simulink model "escooter_sequence_diagram_recuperation"  (R2025b)
settings: Solver=VariableStepAuto  StartTime=0.0  StopTime=10.0  RelTol=1e-3
settings Model: Creator=320236370  LastModifiedBy=320236370

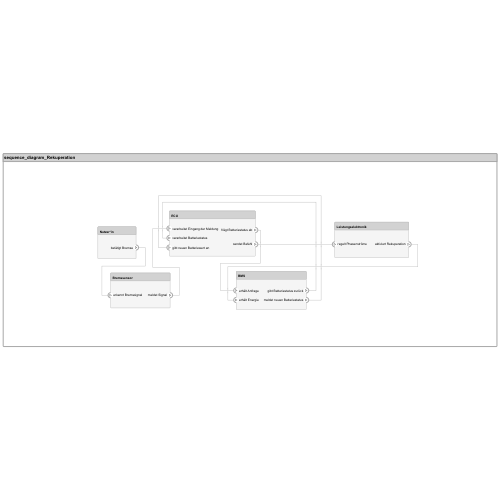
[thumbnail: Simulink's stored preview of the top-level diagram]
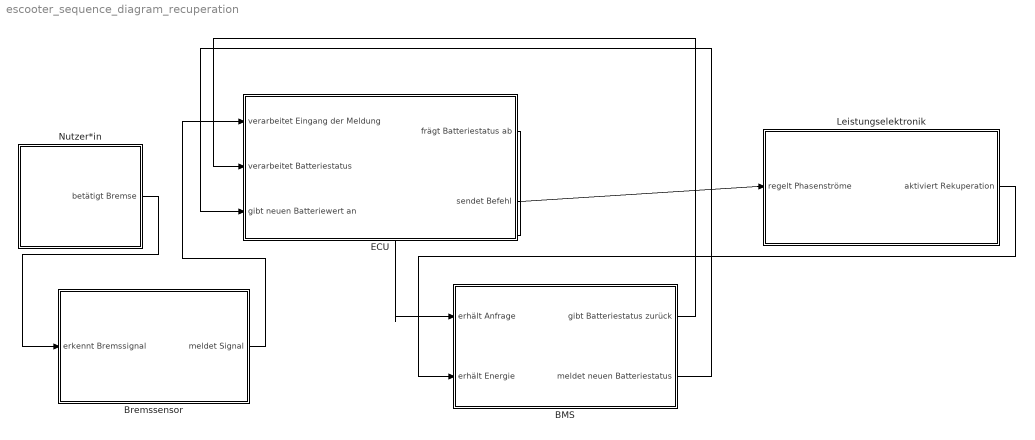
== system escooter_sequence_diagram_recuperation ==
  BMS : Subsystem
      settings: PortSchema="{\"entries\":[{\"content\":{\"headerSize\":26,\"margin\":15,\"minimumSpacing\":25,\"sides\":[{\"content\":{\"connectorIds\":[\"In1\",\"In2\"]},\"type\":\"ConnectorPlacement.EquallySpacedRectSide\",\"uuid\":\"3d49029f-ff69-43f0-9083-eb7baed04898\"},{\"content\":{\"connectorIds\":[\"Out1\",\"Out2\"],\"side\":\"RIGHT\"},\"type\":\"ConnectorPlacement.EquallySpacedRectSide\",\"uuid\":\"1597d90c-c332-40d9-8a70-68f04d256300\"},{\"content\":{\"side\":\"TOP\"},\"type\":\"ConnectorPlacement.EquallySpacedRectSide\",\"uuid\":\"ad895052-9fa6-4dfa-a28f-1843b80a8a3f\"}]},\"type\":\"ConnectorPlacement.EquallySpacedConnector\",\"uuid\":\"8d35fef0-5689-4d8b-850c-97501fa910c2\"}],\"packageUris\":[\"http://schema.mathworks.com/mf0/Connector/R2020b\"],\"version\":\"1.0\"}"
  Bremssensor : Subsystem
      settings: PortSchema="{\"entries\":[{\"content\":{\"headerSize\":26,\"margin\":15,\"minimumSpacing\":25,\"sides\":[{\"content\":{\"connectorIds\":[\"In1\"]},\"type\":\"ConnectorPlacement.EquallySpacedRectSide\",\"uuid\":\"3d49029f-ff69-43f0-9083-eb7baed04898\"},{\"content\":{\"connectorIds\":[\"Out1\"],\"side\":\"RIGHT\"},\"type\":\"ConnectorPlacement.EquallySpacedRectSide\",\"uuid\":\"1597d90c-c332-40d9-8a70-68f04d256300\"},{\"content\":{\"side\":\"TOP\"},\"type\":\"ConnectorPlacement.EquallySpacedRectSide\",\"uuid\":\"ad895052-9fa6-4dfa-a28f-1843b80a8a3f\"}]},\"type\":\"ConnectorPlacement.EquallySpacedConnector\",\"uuid\":\"8d35fef0-5689-4d8b-850c-97501fa910c2\"}],\"packageUris\":[\"http://schema.mathworks.com/mf0/Connector/R2020b\"],\"version\":\"1.0\"}"
  ECU : Subsystem
      settings: PortSchema="{\"entries\":[{\"content\":{\"headerSize\":26,\"margin\":15,\"minimumSpacing\":25,\"sides\":[{\"content\":{\"connectorIds\":[\"In1\",\"In2\",\"In3\"]},\"type\":\"ConnectorPlacement.EquallySpacedRectSide\",\"uuid\":\"3d49029f-ff69-43f0-9083-eb7baed04898\"},{\"content\":{\"connectorIds\":[\"Out1\",\"Out2\"],\"side\":\"RIGHT\"},\"type\":\"ConnectorPlacement.EquallySpacedRectSide\",\"uuid\":\"1597d90c-c332-40d9-8a70-68f04d256300\"},{\"content\":{\"side\":\"TOP\"},\"type\":\"ConnectorPlacement.EquallySpacedRectSide\",\"uuid\":\"ad895052-9fa6-4dfa-a28f-1843b80a8a3f\"}]},\"type\":\"ConnectorPlacement.EquallySpacedConnector\",\"uuid\":\"8d35fef0-5689-4d8b-850c-97501fa910c2\"}],\"packageUris\":[\"http://schema.mathworks.com/mf0/Connector/R2020b\"],\"version\":\"1.0\"}"
  Leistungselektronik : Subsystem
      settings: PortSchema="{\"entries\":[{\"content\":{\"headerSize\":26,\"margin\":15,\"minimumSpacing\":25,\"sides\":[{\"content\":{\"connectorIds\":[\"In1\"]},\"type\":\"ConnectorPlacement.EquallySpacedRectSide\",\"uuid\":\"3d49029f-ff69-43f0-9083-eb7baed04898\"},{\"content\":{\"connectorIds\":[\"Out1\"],\"side\":\"RIGHT\"},\"type\":\"ConnectorPlacement.EquallySpacedRectSide\",\"uuid\":\"1597d90c-c332-40d9-8a70-68f04d256300\"},{\"content\":{\"side\":\"TOP\"},\"type\":\"ConnectorPlacement.EquallySpacedRectSide\",\"uuid\":\"ad895052-9fa6-4dfa-a28f-1843b80a8a3f\"}]},\"type\":\"ConnectorPlacement.EquallySpacedConnector\",\"uuid\":\"8d35fef0-5689-4d8b-850c-97501fa910c2\"}],\"packageUris\":[\"http://schema.mathworks.com/mf0/Connector/R2020b\"],\"version\":\"1.0\"}"
  Nutzer*in : Subsystem
      settings: PortSchema="{\"entries\":[{\"content\":{\"headerSize\":26,\"margin\":15,\"minimumSpacing\":25,\"sides\":[{\"content\":{},\"type\":\"ConnectorPlacement.EquallySpacedRectSide\",\"uuid\":\"3d49029f-ff69-43f0-9083-eb7baed04898\"},{\"content\":{\"connectorIds\":[\"Out1\"],\"side\":\"RIGHT\"},\"type\":\"ConnectorPlacement.EquallySpacedRectSide\",\"uuid\":\"1597d90c-c332-40d9-8a70-68f04d256300\"},{\"content\":{\"side\":\"TOP\"},\"type\":\"ConnectorPlacement.EquallySpacedRectSide\",\"uuid\":\"ad895052-9fa6-4dfa-a28f-1843b80a8a3f\"}]},\"type\":\"ConnectorPlacement.EquallySpacedConnector\",\"uuid\":\"8d35fef0-5689-4d8b-850c-97501fa910c2\"}],\"packageUris\":[\"http://schema.mathworks.com/mf0/Connector/R2020b\"],\"version\":\"1.0\"}"
  wires:
  Nutzer*in/1(betätigt Bremse) -> Bremssensor/1(erkennt Bremssignal)
  Bremssensor/1(meldet Signal) -> ECU/1(verarbeitet Eingang der Meldung)
  ECU/1(frägt Batteriestatus ab) -> BMS/1(erhält Anfrage)
  BMS/1(gibt Batteriestatus zurück) -> ECU/2(verarbeitet Batteriestatus)
  ECU/2(sendet Befehl) -> Leistungselektronik/1(regelt Phasenströme)
  Leistungselektronik/1(aktiviert Rekuperation) -> BMS/2(erhält Energie)
  BMS/2(meldet neuen Batteriestatus) -> ECU/3(gibt neuen Batteriewert an)

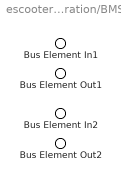
== system escooter_sequence_diagram_recuperation/BMS ==
  Bus Element In1 : Inport  PortName=erhält Anfrage
  Bus Element In2 : Inport  Port=2  PortName=erhält Energie
  Bus Element Out1 : Outport  PortName=gibt Batteriestatus zurück
  Bus Element Out2 : Outport  Port=2  PortName=meldet neuen Batteriestatus

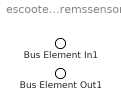
== system escooter_sequence_diagram_recuperation/Bremssensor ==
  Bus Element In1 : Inport  PortName=erkennt Bremssignal
  Bus Element Out1 : Outport  PortName=meldet Signal

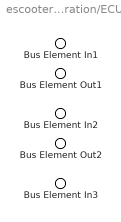
== system escooter_sequence_diagram_recuperation/ECU ==
  Bus Element In1 : Inport  PortName=verarbeitet Eingang der Meldung
  Bus Element In2 : Inport  Port=2  PortName=verarbeitet Batteriestatus
  Bus Element In3 : Inport  Port=3  PortName=gibt neuen Batteriewert an
  Bus Element Out1 : Outport  PortName=frägt Batteriestatus ab
  Bus Element Out2 : Outport  Port=2  PortName=sendet Befehl

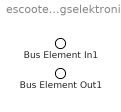
== system escooter_sequence_diagram_recuperation/Leistungselektronik ==
  Bus Element In1 : Inport  PortName=regelt Phasenströme
  Bus Element Out1 : Outport  PortName=aktiviert Rekuperation

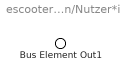
== system escooter_sequence_diagram_recuperation/Nutzer*in ==
  Bus Element Out1 : Outport  PortName=betätigt Bremse
